simulink model "Freq_Spec"  (Simulink 7.3)
settings: Solver=ode45  StartTime=0.0  StopTime=100  RelTol=1e-3
undefined symbols (not defined in the file or in its folder): Fs, get
libraries: dspspect3 x2, dspsnks4 x2, dspbuff3 x1
settings Model: Creator=Peidro  LastModifiedBy=admin
settings DebuggingCC: StrictBusMsg=ErrorLevel1

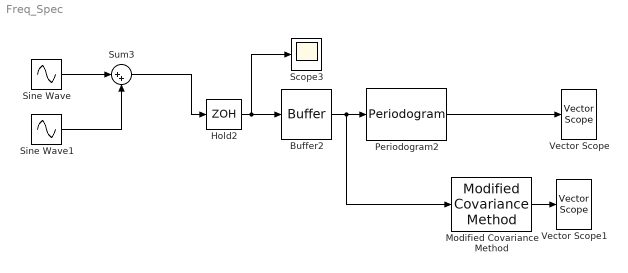
== system Freq_Spec ==
  Buffer2 : dspbuff3/Buffer  N=128  V=64  ic=0
  Hold2 : ZeroOrderHold  SampleTime=0.1
  Modified Covariance Method : dspspect3/Modified Covariance Method  SystemSampleTime=-1  ord=12  inheritFFT=off  fftsize=32
  Periodogram2 : dspspect3/Periodogram  SystemSampleTime=-1  wintype=Hamming  Rs=50  beta=5  winsamp=Periodic  inheritFFT=on  fftsize=128  navg=1
  Scope3 : Scope
      settings: YMin=67.5  YMax=125
  Sine Wave : Sin  Amplitude=1  Bias=0  Frequency=1  Phase=0  Samples=10  SampleTime=0  Offset=0
  Sine Wave1 : Sin  Amplitude=1  Bias=0  Frequency=3  Phase=0  Samples=10  SampleTime=0  Offset=0
  Sum3 : Sum  Inputs=|++  OutDataType=fixdt(1, 16)  OutScaling=2^0
  Vector Scope : dspsnks4/Vector Scope  DialogController=dspdialog.VectorScope  DialogControllerArgs=DataTag0  ScopeProperties=on  Domain=Frequency  HorizSpan=1  DisplayProperties=off  AxisGrid=on  Memory=on  FrameNumber=on  AxisLegend=on  AxisZoom=off  OpenScopeAtSimStart=on  OpenScopeImmediately=off  FigPos=get(0,'defaultfigureposition')  AxisProperties=off  XUnits=rad/sec  XRange=[-Fs/2...Fs/2]  InheritXIncr=on  XIncr=1  XLabel=Time  XLimit=Auto  XMin=0  XMax=0.5  XStart=0  YUnits=dB  YLabel=Amplitude  LineProperties=off  LineColors=[1 0 0]|[0 0 1]  XAxisParamsVer=6.9
      settings: YMin=-30.4175  YMax=59.7698
  Vector Scope1 : dspsnks4/Vector Scope  DialogController=dspdialog.VectorScope  DialogControllerArgs=DataTag1  ScopeProperties=on  Domain=Frequency  HorizSpan=1  DisplayProperties=off  AxisGrid=on  Memory=on  FrameNumber=on  AxisLegend=on  AxisZoom=off  OpenScopeAtSimStart=on  OpenScopeImmediately=off  FigPos=get(0,'defaultfigureposition')  AxisProperties=off  XUnits=rad/sec  XRange=[0...Fs]  InheritXIncr=on  XIncr=1  XLabel=Time  XLimit=Auto  XMin=0  XMax=0.5  XStart=0  YUnits=dB  YLabel=Amplitude  LineProperties=off  LineColors=[1 0 0]|[0 0 1]  XAxisParamsVer=6.9
      settings: YMin=-30.4175  YMax=59.7698
  wires:
  Periodogram2/1 -> Vector Scope/1
  Hold2/1 -> Buffer2/1, Scope3/1
  Buffer2/1 -> Periodogram2/1, Modified Covariance Method/1
  Sine Wave/1 -> Sum3/1
  Sine Wave1/1 -> Sum3/2
  Sum3/1 -> Hold2/1
  Modified Covariance Method/1 -> Vector Scope1/1
